simulink subsystem "Electrode_Hydraulic"  (R2025b)
settings: Solver=VariableStepAuto  StartTime=0.0  StopTime=10.0  RelTol=1e-3
values from neighbouring files (symbols this model uses):
  Ts_ctrl = 5e-3    (= 0.005)    [ctrlSys_init.m]
undefined symbols (not defined in the file or in its folder): k
settings Model: Creator=LYG  LastModifiedBy=LYG

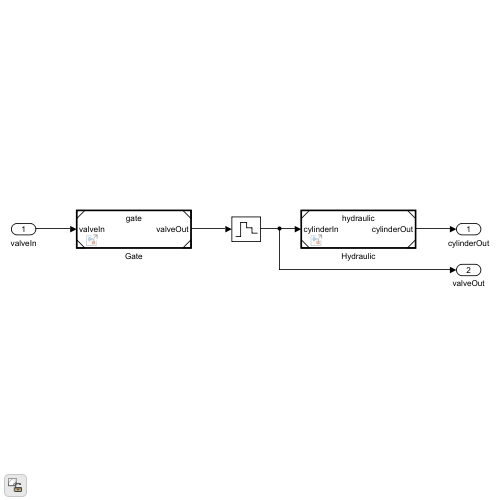
[thumbnail: Simulink's stored preview of the top-level diagram]
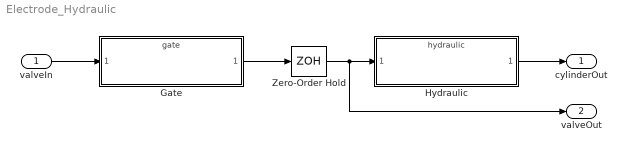
== system Electrode_Hydraulic ==
  valveIn : Inport
  Gate : ModelReference  ModelNameDialog=gate.slx  UsingDefaultArgumentValue=0,0,0,0,0,0,0  SimulationMode=Normal  ModelReferenceVersion=3.2  Ksvr=Ksvr  Ksvl=Ksvl  Xmax=Xmax  Xmin=Xmin  dl=dl  dr=dr  k=k
  Hydraulic : ModelReference  ModelNameDialog=hydraulic.slx  UsingDefaultArgumentValue=0,0,0,0,0,0,0,0,0  SimulationMode=Normal  ModelReferenceVersion=3.6  Ap=Ap  Ct=Ct  Fforce=Fforce  Gmass=Gmass  Kc=Kc  Kq=Kq  Ve=Ve  beta_e=beta_e  L_init=L_init
  Zero-Order Hold : ZeroOrderHold  SampleTime=Ts_ctrl
  cylinderOut : Outport
  valveOut : Outport  Port=2
  wires:
  Hydraulic/1 -> cylinderOut/1
  valveIn/1 -> Gate/1
  Gate/1 -> Zero-Order Hold/1
  Zero-Order Hold/1 -> Hydraulic/1, valveOut/1
